simulink model "Project_Vehicle_Model_Round_One"  (R2018b)
settings: Solver=VariableStepAuto  StartTime=0  StopTime=1923  MaxStep=0.01  RelTol=1e-3
values from neighbouring files (symbols this model uses):
  A_CS = 12    [Project_Round_One.m]
  C_D = 0.36    [Project_Round_One.m]
  F_RR = f_RR * mass_total * g * cos(beta)    [Project_Round_One.m]
  F_slope = mass_total * g * sin(beta)    [Project_Round_One.m]
  mass_total = mass_veh + mass_payload + mass_batt + mass_motor    (= 18769)    [Project_Round_One.m]
  P_aux = 10    [Project_Round_One.m]
  RHO = 1.17    [Project_Round_One.m]
  speed_m_s = speed_km_h .* (5/18)    [Project_Round_One.m]
  trans_eff = 0.9    [Project_Round_One.m]
libraries: simulink x1
settings Model: Creator=tammik2  LastModifiedBy=subhadyutisahoo
settings DebuggingCC: LibraryContextMissingDiagnostic=none
settings SFSimCC: SimUseLocalCustomCode=off
settings RTWCC: RTWUseLocalCustomCode=off
settings CodeAppCC: StateflowObjectComments=on

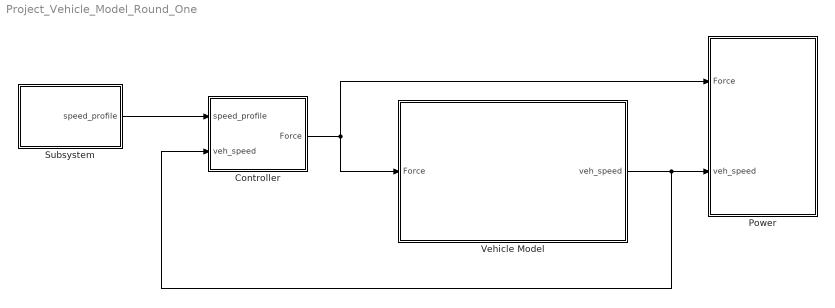
== system Project_Vehicle_Model_Round_One ==
  Controller : Subsystem
  Power : Subsystem
  Subsystem : Subsystem
  Vehicle Model : Subsystem
  wires:
  Controller/1(Force) -> Power/1(Force), Vehicle Model/1(Force)
  Vehicle Model/1(veh_speed) -> Controller/2(veh_speed), Power/2(veh_speed)
  Subsystem/1(speed_profile) -> Controller/1(speed_profile)

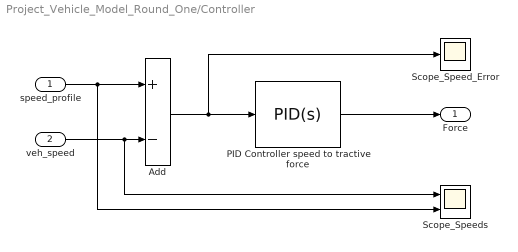
== system Project_Vehicle_Model_Round_One/Controller ==
  speed_profile : Inport
  veh_speed : Inport  Port=2
  Add : Sum  Inputs=+-
  PID Controller speed to tractive force : simulink/Continuous/PID Controller  Controller=PID  Form=Parallel  TimeDomain=Continuous-time  SampleTime=-1  IntegratorMethod=Forward Euler  FilterMethod=Forward Euler  ControllerParametersSource=internal  P=1978.20669524817  I=378.395999263715  D=-416.880241054576  UseFilter=on  N=1.72044274974478  TunerSelectOption=Transfer Function Based (PID Tuner App)  InitialConditionSource=internal  InitialConditionForIntegrator=0  InitialConditionForFilter=0  DifferentiatorICPrevScaledInput=0  ExternalReset=none  TrackingMode=off  Kt=1  LimitOutput=off  UpperSaturationLimit=inf  LowerSaturationLimit=-inf  LinearizeAsGain=on  AntiWindupMode=none  Kb=1  POutMin=[]  POutMax=[]  IOutMin=[]  IOutMax=[]  DOutMin=[]  DOutMax=[]  NOutMin=[]  NOutMax=[]  SumOutMin=[]  SumOutMax=[]  SaturationOutMin=[]  SaturationOutMax=[]  PParamMin=[]  PParamMax=[]  IParamMin=[]  IParamMax=[]  DParamMin=[]  DParamMax=[]  NParamMin=[]  NParamMax=[]  KbParamMin=[]  KbParamMax=[]  KtParamMin=[]  KtParamMax=[]  KbOutMin=[]  KbOutMax=[]  KtOutMin=[]  KtOutMax=[]  IntegratorOutMin=[]  IntegratorOutMax=[]  FilterOutMin=[]  FilterOutMax=[]  SumI1OutMin=[]  SumI1OutMax=[]  SumI2OutMin=[]  SumI2OutMax=[]  SumI3OutMin=[]  SumI3OutMax=[]  SumI4OutMin=[]  SumI4OutMax=[]  SumDOutMin=[]  SumDOutMax=[]  DifferentiatorOutMin=[]  DifferentiatorOutMax=[]  FilterDiffOutCoefMin=[]  FilterDiffOutCoefMax=[]  ReciprocalOutMin=[]  ReciprocalOutMax=[]  SumDenOutMin=[]  SumDenOutMax=[]  SumNumOutMin=[]  SumNumOutMax=[]  DivideOutMin=[]  DivideOutMax=[]  IntegratorContinuousStateAttributes=''  IntegratorStateMustResolveToSignalObject=off  IntegratorRTWStateStorageClass=Auto  FilterContinuousStateAttributes=''  FilterStateMustResolveToSignalObject=off  FilterRTWStateStorageClass=Auto  ParallelPVariant=InternalParameters  IdealPVariant=Disabled  IVariant=InternalParameters  DVariant=InternalParameters  IntegratorVariant=Continuous  SatVariant=Disabled  AWVariant=Passthrough  PCopyVariant=Disabled  TRVariant=Disabled  FdbkBlocksVariant=Forward  IdealPFdbkVariant=Disabled  SatFdbkVariant=Disabled  DerivativeFilterVariant=ContFilter  NVariant=InternalParameters  NCopyVariant=Disabled  FilterICVariant=InternalICsFilter  IntegratorICVariant=InternalICs  ExternalResetVariant=Disabled  TRSumVariant=Passthrough  SumFdbkVariant=Disabled  SumVariant=Sum_PID
  "Scope_Speed_Error " : Scope
  Scope_Speeds : Scope  NumInputPorts=2
  Force : Outport
  wires:
  veh_speed/1 -> Scope_Speeds/1, Add/2
  speed_profile/1 -> Scope_Speeds/2, Add/1
  Add/1 -> "Scope_Speed_Error "/1, PID Controller speed to tractive force/1
  PID Controller speed to tractive force/1 -> Force/1

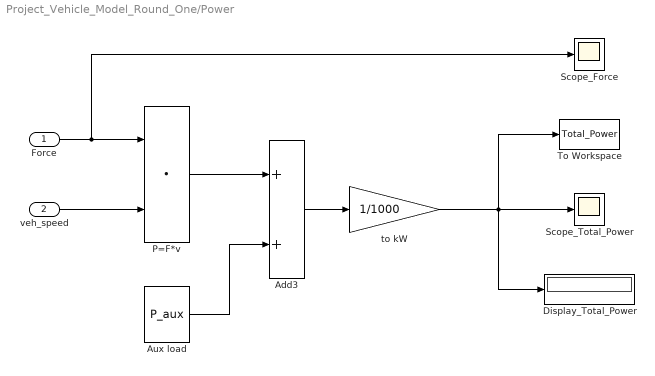
== system Project_Vehicle_Model_Round_One/Power ==
  Force : Inport
  veh_speed : Inport  Port=2
  Add3 : Sum
  Aux load : Constant  Value=P_aux
  Display_Total_Power : Display
  P=F*v : DotProduct  InputSameDT=on  OutDataTypeStr=Inherit: Inherit via internal rule
  Scope_Force : Scope
  Scope_Total_Power : Scope
  To Workspace : ToWorkspace  VariableName=Total_Power  SaveFormat=Timeseries  SampleTime=-1
  to kW : Gain  Gain=1/1000
  wires:
  veh_speed/1 -> P=F*v/2
  Force/1 -> Scope_Force/1, P=F*v/1
  P=F*v/1 -> Add3/1
  Aux load/1 -> Add3/2
  Add3/1 -> to kW/1
  to kW/1 -> Display_Total_Power/1, To Workspace/1, Scope_Total_Power/1

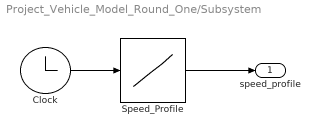
== system Project_Vehicle_Model_Round_One/Subsystem ==
  Clock : Clock
  Speed_Profile : Lookup_n-D  NumberOfTableDimensions=1  BreakpointsSpecification=Even spacing  BreakpointsForDimension1=[0:1923]  Table=speed_m_s  InternalRulePriority=Speed  RndMeth=Simplest  InputSameDT=on
  speed_profile : Outport
  wires:
  Speed_Profile/1 -> speed_profile/1
  Clock/1 -> Speed_Profile/1

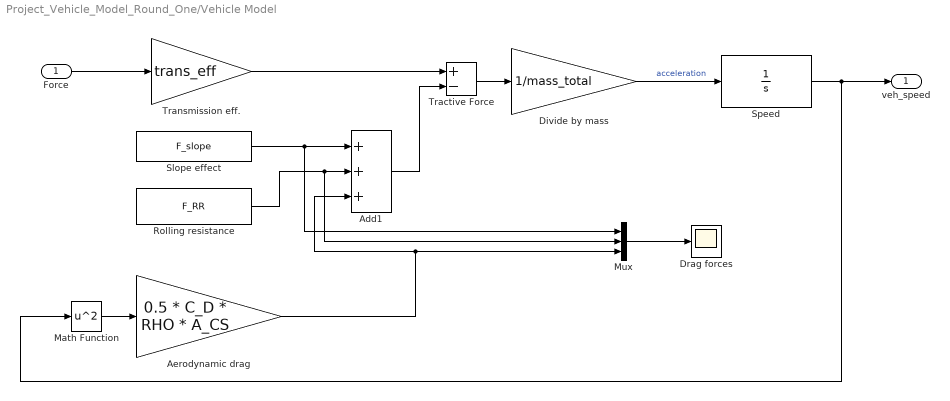
== system Project_Vehicle_Model_Round_One/Vehicle Model ==
  Force : Inport
  Add1 : Sum  Inputs=+++
  Aerodynamic drag : Gain  Gain=0.5 * C_D * RHO * A_CS
  "Divide by mass " : Gain  Gain=1/mass_total
  Drag forces : Scope
  Math Function : Math  Operator=square  SaturateOnIntegerOverflow=on
  Mux : Mux  Inputs=3
  Rolling resistance : Constant  Value=F_RR
  Slope effect : Constant  Value=F_slope
  Speed : TransferFcn  Denominator=[1 0]
  Tractive Force : Sum  Inputs=+-
  Transmission eff. : Gain  Gain=trans_eff
  veh_speed : Outport
  wires:
  Speed/1 -> Math Function/1, veh_speed/1
  Force/1 -> Transmission eff./1
  Rolling resistance/1 -> Mux/2, Add1/2
  "Divide by mass "/1 -> Speed/1  "acceleration"
  Add1/1 -> Tractive Force/2
  Math Function/1 -> Aerodynamic drag/1
  Transmission eff./1 -> Tractive Force/1
  Aerodynamic drag/1 -> Add1/3, Mux/3
  Mux/1 -> Drag forces/1
  Tractive Force/1 -> "Divide by mass "/1
  Slope effect/1 -> Mux/1, Add1/1
